simulink model "PHIL_SF3_egston_adapted"  (R2016a)
settings: Solver=FixedStepAuto  StartTime=0.0  StopTime=10.0  FixedStep=0.0002  RelTol=1e-3
settings Model: Creator=CoSES_HPC2  LastModifiedBy=CoSES_HPC2
settings DebuggingCC: RootOutportRequireBusObject=error  StrictBusMsg=ErrorOnBusTreatedAsVector
settings HardwareCC: ProdBitPerPointer=32  ProdLargestAtomicFloat=None  ProdWordSize=32  ProdHWDeviceType=Intel->x86/Pentium
settings RTWCC: SystemTargetFile=NIVeriStand.tlc  TemplateMakefile=NIVeriStand_vc.tmf  Description=NI Phar Lap Real-Time & Windows Targets
settings STFCustomTargetCC: MatFileLogging=on  SystemTargetFile=NIVeriStand.tlc
settings GRTTargetCC: ParMdlRefBuildCompliant=off  CompOptLevelCompliant=off  ConcurrentExecutionCompliant=off  GeneratePreprocessorConditionals=Use local settings  CombineOutputUpdateFcns=off  CPPClassGenCompliant=off  GRTInterface=on  UseToolchainInfoCompliant=off

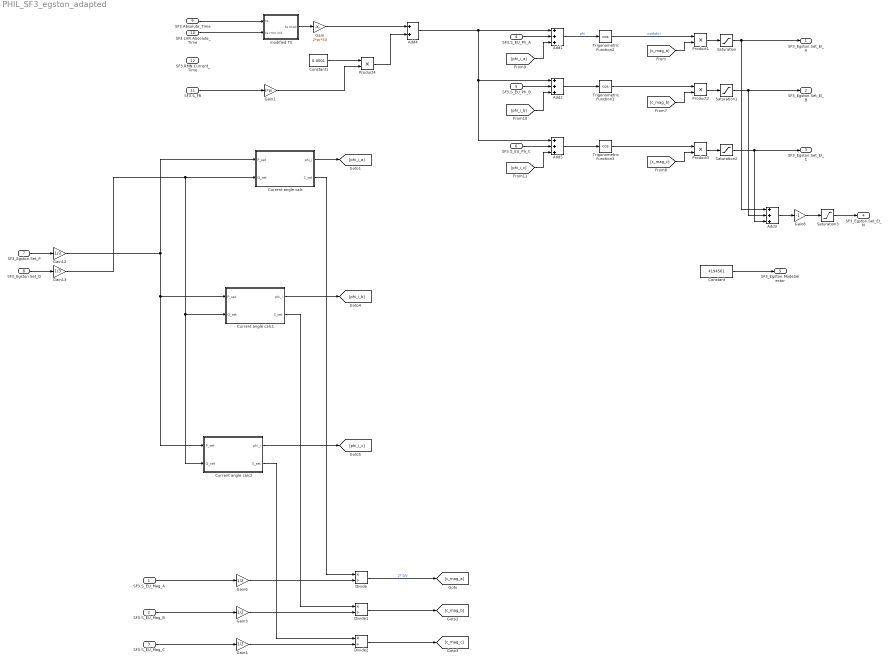
== system PHIL_SF3_egston_adapted ==
  SF3.S_EU_Mag_A : Inport
  SF3.S_EU_Mag_B : Inport  Port=2
  SF3.S_EU_Mag_C : Inport  Port=3
  SF3.S_EU_Ph_A : Inport  Port=4
  SF3.S_EU_Ph_B : Inport  Port=5
  SF3.S_EU_Ph_C : Inport  Port=6
  SF3_Egston.Set_P : Inport  Port=7
  SF3_Egston.Set_Q : Inport  Port=8
  SF3.Absolute_Time : Inport  Port=9
  SF3.LVR.Absolute_Time : Inport  Port=10
  SF3.S_FR : Inport  Port=11
  SF3.RMN.Current_Time : Inport  Port=12
  Add{1..3,5} (4 alike) : Sum  Inputs=+++
  Add4 : Sum
  Constant : Constant  Value=4194561
  Constant1 : Constant  Value=0.0001
  Current angle calc : Subsystem
  Current angle calc1 : Subsystem
  Current angle calc2 : Subsystem
  Divide : Product  Inputs=*/
  Divide1 : Product  Inputs=*/
  Divide2 : Product  Inputs=*/
  Gain : Gain  Gain=2*pi*50
  Gain1 : Gain  Gain=2*pi
  Gain12 : Gain  Gain=1/3
  Gain13 : Gain  Gain=1/3
  Gain3 : Gain  Gain=1/2
  Gain4 : Gain  Gain=1/2
  Gain6 : Gain  Gain=1/2
  Gain8 : Gain  Gain=-1
  Product{1..4} (4 alike) : Product
  Saturation{,1..3} (4 alike) : Saturate  UpperLimit=100  LowerLimit=-100
  Trigonometric Function1 : Trigonometry  Operator=cos
  Trigonometric Function2 : Trigonometry  Operator=cos
  Trigonometric Function3 : Trigonometry  Operator=cos
  modified TS : Subsystem
  SF3_Egston.Set_EI_A : Outport
  SF3_Egston.Set_EI_B : Outport  Port=2
  SF3_Egston.Set_EI_C : Outport  Port=3
  SF3_Egston.Set_EI_N : Outport  Port=4
  SF3_Egston.ModeSelector : Outport  Port=5
  wires:
  Trigonometric Function2/1 -> Product1/1  "cos(phi)"
  Trigonometric Function1/1 -> Product2/1
  Trigonometric Function3/1 -> Product3/1
  Add1/1 -> Trigonometric Function2/1  "phi"
  Add2/1 -> Trigonometric Function1/1
  Add5/1 -> Trigonometric Function3/1
  [c_mag_a] -> Product1/2
  [c_mag_b] -> Product2/2
  [c_mag_c] -> Product3/2
  SF3.S_EU_Ph_C/1 -> Add5/2
  SF3.S_EU_Ph_B/1 -> Add2/2
  [phi_i_a] -> Add1/3
  [phi_i_b] -> Add2/3
  [phi_i_c] -> Add5/3
  Product1/1 -> Saturation/1
  Product2/1 -> Saturation1/1
  Product3/1 -> Saturation2/1
  SF3.S_EU_Ph_A/1 -> Add1/2
  Current angle calc/1(phi_i) -> [phi_i_a]
  SF3.S_EU_Mag_A/1 -> Gain6/1
  SF3.S_EU_Mag_B/1 -> Gain3/1
  SF3.S_EU_Mag_C/1 -> Gain4/1
  Divide/1 -> [c_mag_a]  "2? S/V"
  Divide1/1 -> [c_mag_b]
  Divide2/1 -> [c_mag_c]
  Gain6/1 -> Divide/2
  Gain3/1 -> Divide1/2
  Gain4/1 -> Divide2/2
  Saturation/1 -> Add3/1, SF3_Egston.Set_EI_A/1
  Saturation1/1 -> SF3_Egston.Set_EI_B/1, Add3/2
  Saturation2/1 -> SF3_Egston.Set_EI_C/1, Add3/3
  Add3/1 -> Gain8/1
  Gain8/1 -> Saturation3/1
  Current angle calc1/1(phi_i) -> [phi_i_b]
  Current angle calc2/1(phi_i) -> [phi_i_c]
  Current angle calc/2(S_set) -> Divide/1
  Current angle calc1/2(S_set) -> Divide1/1
  Current angle calc2/2(S_set) -> Divide2/1
  Saturation3/1 -> SF3_Egston.Set_EI_N/1
  SF3_Egston.Set_P/1 -> Gain12/1
  SF3_Egston.Set_Q/1 -> Gain13/1
  Gain12/1 -> Current angle calc/1(P_set), Current angle calc2/1(P_set), Current angle calc1/1(P_set)
  Gain13/1 -> Current angle calc2/2(Q_set), Current angle calc1/2(Q_set), Current angle calc/2(Q_set)
  SF3.Absolute_Time/1 -> modified TS/1(ts)
  SF3.LVR.Absolute_Time/1 -> modified TS/2(ts rmn init)
  modified TS/1(ts mod) -> Gain/1
  Constant1/1 -> Product4/1
  Gain/1 -> Add4/1
  Product4/1 -> Add4/2
  SF3.S_FR/1 -> Gain1/1
  Gain1/1 -> Product4/2
  Add4/1 -> Add1/1, Add5/1, Add2/1
  Constant/1 -> SF3_Egston.ModeSelector/1

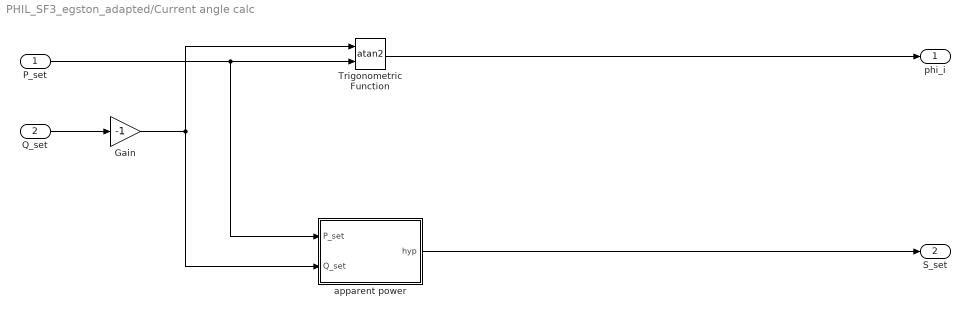
== system PHIL_SF3_egston_adapted/Current angle calc ==
  P_set : Inport
  Q_set : Inport  Port=2
  Gain : Gain  Gain=-1
  Trigonometric Function : Trigonometry  Operator=atan2
  apparent power : Subsystem
  phi_i : Outport
  S_set : Outport  Port=2
  wires:
  P_set/1 -> Trigonometric Function/2, apparent power/1(P_set)
  Q_set/1 -> Gain/1
  apparent power/1(hyp) -> S_set/1
  Trigonometric Function/1 -> phi_i/1
  Gain/1 -> apparent power/2(Q_set), Trigonometric Function/1

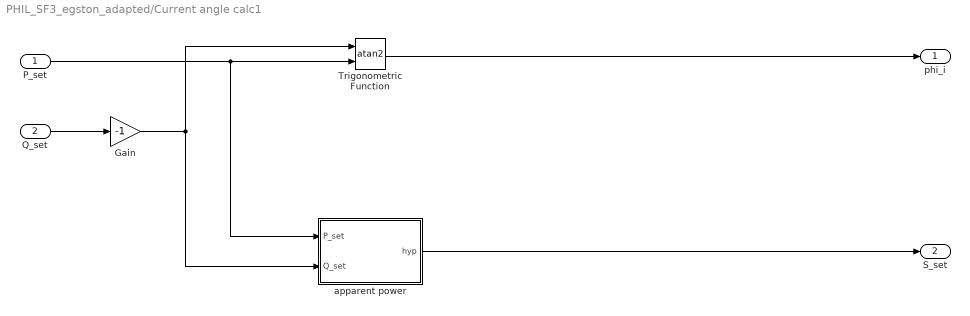
== system PHIL_SF3_egston_adapted/Current angle calc1 ==
  P_set : Inport
  Q_set : Inport  Port=2
  Gain : Gain  Gain=-1
  Trigonometric Function : Trigonometry  Operator=atan2
  apparent power : Subsystem
  phi_i : Outport
  S_set : Outport  Port=2
  wires:
  P_set/1 -> Trigonometric Function/2, apparent power/1(P_set)
  Q_set/1 -> Gain/1
  apparent power/1(hyp) -> S_set/1
  Trigonometric Function/1 -> phi_i/1
  Gain/1 -> apparent power/2(Q_set), Trigonometric Function/1

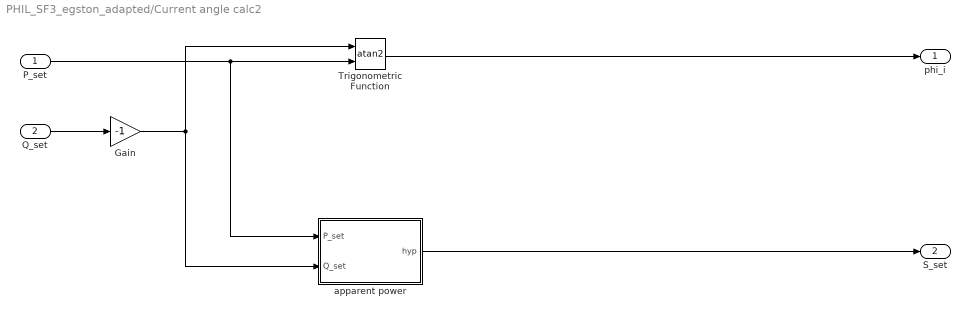
== system PHIL_SF3_egston_adapted/Current angle calc2 ==
  P_set : Inport
  Q_set : Inport  Port=2
  Gain : Gain  Gain=-1
  Trigonometric Function : Trigonometry  Operator=atan2
  apparent power : Subsystem
  phi_i : Outport
  S_set : Outport  Port=2
  wires:
  P_set/1 -> Trigonometric Function/2, apparent power/1(P_set)
  Q_set/1 -> Gain/1
  apparent power/1(hyp) -> S_set/1
  Trigonometric Function/1 -> phi_i/1
  Gain/1 -> apparent power/2(Q_set), Trigonometric Function/1

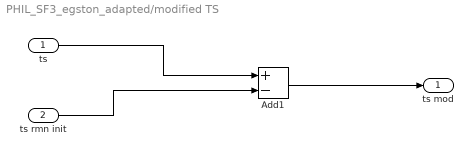
== system PHIL_SF3_egston_adapted/modified TS ==
  ts : Inport
  ts rmn init : Inport  Port=2
  Add1 : Sum  Inputs=+-
  ts mod : Outport
  wires:
  Add1/1 -> ts mod/1
  ts rmn init/1 -> Add1/2
  ts/1 -> Add1/1

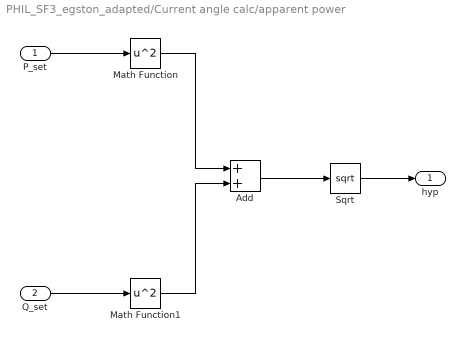
== system PHIL_SF3_egston_adapted/Current angle calc/apparent power ==
  P_set : Inport
  Q_set : Inport  Port=2
  Add : Sum
  Math Function : Math  Operator=square  SaturateOnIntegerOverflow=on
  Math Function1 : Math  Operator=square  SaturateOnIntegerOverflow=on
  Sqrt : Sqrt  SaturateOnIntegerOverflow=on
  hyp : Outport
  wires:
  P_set/1 -> Math Function/1
  Q_set/1 -> Math Function1/1
  Math Function/1 -> Add/1
  Math Function1/1 -> Add/2
  Add/1 -> Sqrt/1
  Sqrt/1 -> hyp/1

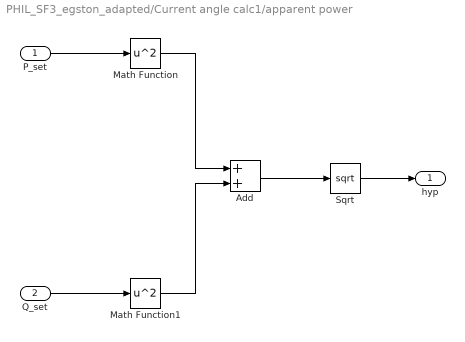
== system PHIL_SF3_egston_adapted/Current angle calc1/apparent power ==
  P_set : Inport
  Q_set : Inport  Port=2
  Add : Sum
  Math Function : Math  Operator=square  SaturateOnIntegerOverflow=on
  Math Function1 : Math  Operator=square  SaturateOnIntegerOverflow=on
  Sqrt : Sqrt  SaturateOnIntegerOverflow=on
  hyp : Outport
  wires:
  P_set/1 -> Math Function/1
  Q_set/1 -> Math Function1/1
  Math Function/1 -> Add/1
  Math Function1/1 -> Add/2
  Add/1 -> Sqrt/1
  Sqrt/1 -> hyp/1

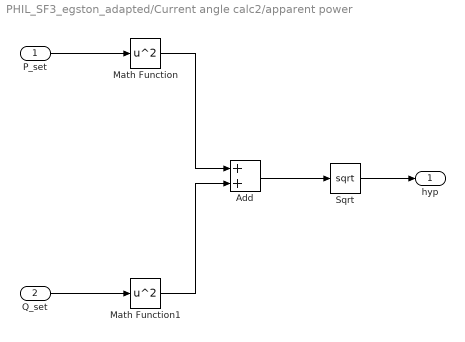
== system PHIL_SF3_egston_adapted/Current angle calc2/apparent power ==
  P_set : Inport
  Q_set : Inport  Port=2
  Add : Sum
  Math Function : Math  Operator=square  SaturateOnIntegerOverflow=on
  Math Function1 : Math  Operator=square  SaturateOnIntegerOverflow=on
  Sqrt : Sqrt  SaturateOnIntegerOverflow=on
  hyp : Outport
  wires:
  P_set/1 -> Math Function/1
  Q_set/1 -> Math Function1/1
  Math Function/1 -> Add/1
  Math Function1/1 -> Add/2
  Add/1 -> Sqrt/1
  Sqrt/1 -> hyp/1
